simulink model "Aufgabe3_sim"  (R2023b)
settings: Solver=VariableStepAuto  StartTime=0.0  StopTime=10.0  RelTol=1e-3
values from neighbouring files (symbols this model uses):
  C2 = 1e-7    (= 1e-07)    [Aufgabe_3_Parameter.m]
  C3 = 1e-9    (= 1e-09)    [Aufgabe_3_Parameter.m]
  gewicht = 5    [Aufgabe_3_Parameter.m]
  K1 = 1    [Aufgabe_3_Parameter.m]
  K2 = 1    [Aufgabe_3_Parameter.m]
  K3 = 1    [Aufgabe_3_Parameter.m]
  R2 = 10e3    (= 10000)    [Aufgabe_3_Parameter.m]
  R3 = 10e3    (= 10000)    [Aufgabe_3_Parameter.m]
  R4 = 1e3    (= 1000)    [Aufgabe_3_Parameter.m]
  R5 = 10e3    (= 10000)    [Aufgabe_3_Parameter.m]
  R6 = 2e3    (= 2000)    [Aufgabe_3_Parameter.m]
  T1 = 1e-3    (= 0.001)    [Aufgabe_3_Parameter.m]
  T2 = 0.75e-3    (= 0.00075)    [Aufgabe_3_Parameter.m]
  T3 = 0.5e-3    (= 0.0005)    [Aufgabe_3_Parameter.m]
settings Model: Creator=Rouven Harmgarth  LastModifiedBy=danie

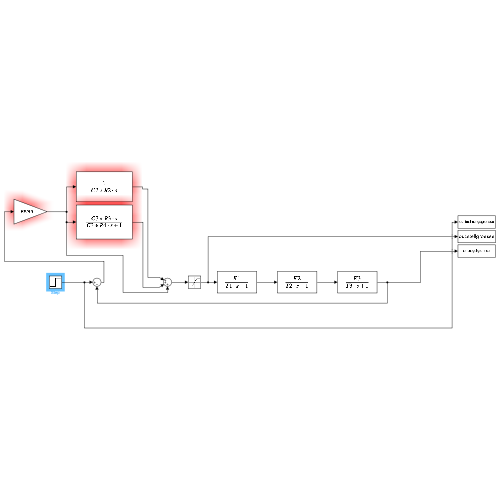
[thumbnail: Simulink's stored preview of the top-level diagram]
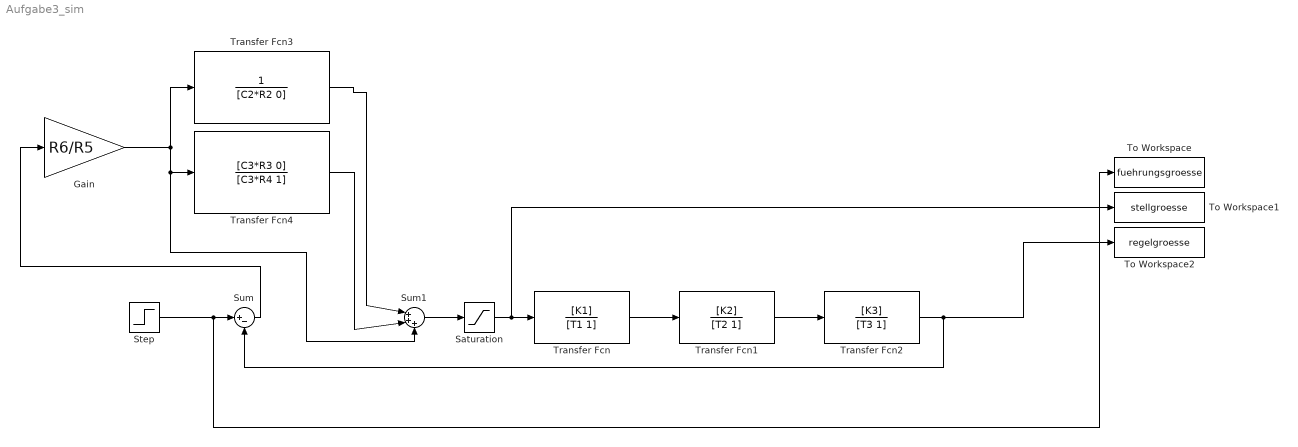
== system Aufgabe3_sim ==
  Gain : Gain  Gain=R6/R5
  Saturation : Saturate  UpperLimit=12  LowerLimit=-12
  Step : Step  Time=0  After=gewicht  SampleTime=0
  Sum : Sum  Inputs=|+-
  Sum1 : Sum  Inputs=|+++
  To Workspace : ToWorkspace  VariableName=fuehrungsgroesse  SaveFormat=Structure With Time  SampleTime=-1
  To Workspace1 : ToWorkspace  VariableName=stellgroesse  SaveFormat=Structure With Time  SampleTime=-1
  To Workspace2 : ToWorkspace  VariableName=regelgroesse  SaveFormat=Structure With Time  SampleTime=-1
  Transfer Fcn : TransferFcn  Numerator=[K1]  Denominator=[T1 1]
  Transfer Fcn1 : TransferFcn  Numerator=[K2]  Denominator=[T2 1]
  Transfer Fcn2 : TransferFcn  Numerator=[K3]  Denominator=[T3 1]
  Transfer Fcn3 : TransferFcn  Denominator=[C2*R2 0]
  Transfer Fcn4 : TransferFcn  Numerator=[C3*R3 0]  Denominator=[C3*R4 1]
  wires:
  Transfer Fcn/1 -> Transfer Fcn1/1
  Transfer Fcn1/1 -> Transfer Fcn2/1
  Saturation/1 -> To Workspace1/1, Transfer Fcn/1
  Step/1 -> To Workspace/1, Sum/1
  Transfer Fcn2/1 -> To Workspace2/1, Sum/2
  Sum/1 -> Gain/1
  Gain/1 -> Sum1/3, Transfer Fcn4/1, Transfer Fcn3/1
  Transfer Fcn4/1 -> Sum1/2
  Transfer Fcn3/1 -> Sum1/1
  Sum1/1 -> Saturation/1
